simulink model "Motor_model"  (R2021b)
settings: Solver=VariableStepAuto  StartTime=0.0  StopTime=10  RelTol=1e-3
values from neighbouring files (symbols this model uses):
  B = 0.02    [Motor_Model.m]
  J = 5    [Motor_Model.m]
  K = 1.4    [Motor_Model.m]
  La = 0.016    [Motor_Model.m]
  Ra = 0.78    [Motor_Model.m]
  T1 = 30    [Motor_Model.m]
settings Model: Creator=user  LastModifiedBy=mahya
settings SolverCC: AlgebraicLoopSolver=TrustRegion
settings DataIOCC: ReturnWorkspaceOutputs=off
settings DebuggingCC: SFMachineParentedDataDiag=warning  ArithmeticOperatorsInVariantConditions=warning
settings SFSimCC: CustomCodeUndefinedFunction=UseInterfaceOnly

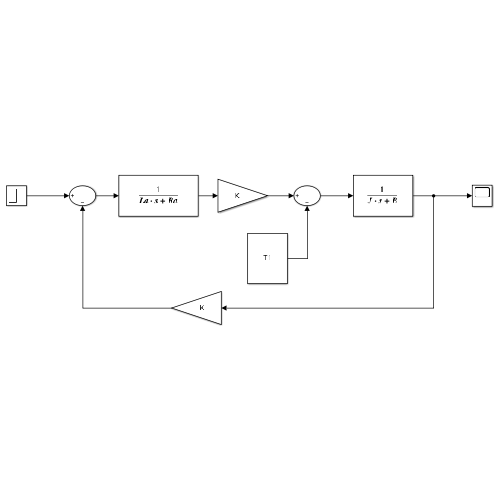
[thumbnail: Simulink's stored preview of the top-level diagram]
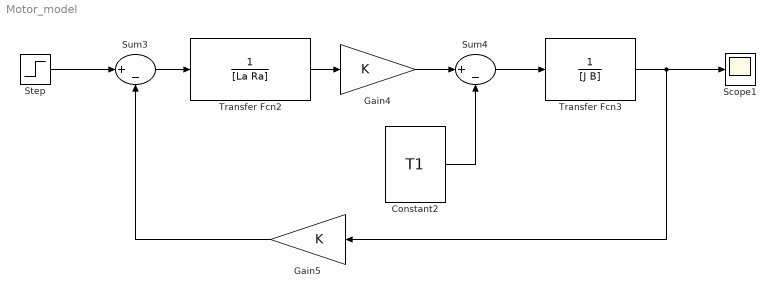
== system Motor_model ==
  Constant2 : Constant  Value=T1
  Gain4 : Gain  Gain=K
  Gain5 : Gain  Gain=K
  Scope1 : Scope
  Step : Step  After=240  SampleTime=0
  Sum3 : Sum  Inputs=|+-
  Sum4 : Sum  Inputs=|+-
  Transfer Fcn2 : TransferFcn  Denominator=[La Ra]
  Transfer Fcn3 : TransferFcn  Denominator=[J B]
  wires:
  Gain5/1 -> Sum3/2
  Constant2/1 -> Sum4/2
  Sum3/1 -> Transfer Fcn2/1
  Gain4/1 -> Sum4/1
  Sum4/1 -> Transfer Fcn3/1
  Transfer Fcn2/1 -> Gain4/1
  Transfer Fcn3/1 -> Scope1/1, Gain5/1
  Step/1 -> Sum3/1
